simulink model "dynamic"  (R2023b)
settings: Solver=VariableStepAuto  StartTime=0.0  StopTime=5  MaxStep=1e-5  RelTol=1e-3
values from neighbouring files (symbols this model uses):
  phi0 = 0    [main.m]
  phidot0 = 0    [main.m]
  psif0 = 0    [main.m]
  psifdot0 = 0    [main.m]
  psir0 = 0    [main.m]
  psirdot0 = 0    [main.m]
  rho0 = 0    [main.m]
  rhodot0 = 0    [main.m]
  theta_dot_fl0 = xdot0*cos(car.toe.fl*pi/180)/car.tr.fl    [main.m]
  theta_dot_fr0 = xdot0*cos(car.toe.fr*pi/180)/car.tr.fr    [main.m]
  theta_dot_rl0 = xdot0*cos(car.toe.rl*pi/180)/car.tr.rl    [main.m]
  theta_dot_rr0 = xdot0*cos(car.toe.rr*pi/180)/car.tr.rr    [main.m]
  x0 = 0    [main.m]
  xdot0 = 10    [main.m]
  y0 = 0    [main.m]
  ydot0 = 0    [main.m]
  Zs0 = 0    [main.m]
  Zsdot0 = 0    [main.m]
  Zufl0 = 0    [main.m]
  Zufldot0 = 0    [main.m]
  Zufr0 = 0    [main.m]
  Zufrdot0 = 0    [main.m]
  Zurl0 = 0    [main.m]
  Zurldot0 = 0    [main.m]
  Zurr0 = 0    [main.m]
  Zurrdot0 = 0    [main.m]
undefined symbols (not defined in the file or in its folder): car
libraries: simulink x4, spsFirstOrderFilterLib x1
(part 2 of 2)

== system dynamic/Roll, Pitch, Heave/Unsprung/Unsprung rl ==
  Zf : Inport
  Z0 : Inport  Port=2
  Bus Creator : BusCreator  Inputs=3
  Bus Selector : BusSelector  OutputSignals=Zf_rl
  Bus Selector1 : BusSelector  OutputSignals=Z0_rl,Z0dot_rl
  Constant : Constant  Value=car.g
  Gain : Gain  Gain=car.K.t
  Gain1 : Gain  Gain=car.c.t
  Gain2 : Gain  Gain=1/car.murl
  Gain4 : Gain  Gain=car.murl
  Integrator : Integrator  InitialCondition=Zurldot0
  Integrator1 : Integrator  InitialCondition=Zurl0
  Minus : Sum  Inputs=----
  Minus1 : Sum  Inputs=+-
  Minus2 : Sum  Inputs=+-
  Minus3 : Sum
  Zu_rl : Outport
  FZ_rl : Outport  Port=2
  wires:
  Z0/1 -> Bus Selector1/1
  Zf/1 -> Bus Selector/1
  Bus Selector/1 -> Minus/1  "<Zf_rl>"
  Bus Selector1/1 -> Minus1/2  "<Z0_rl>"
  Minus1/1 -> Gain/1
  Gain/1 -> Minus/2, Minus3/1
  Bus Selector1/2 -> Minus2/2  "<Z0dot_rl>"
  Minus2/1 -> Gain1/1
  Gain1/1 -> Minus/3, Minus3/2
  Minus/1 -> Gain2/1
  Gain2/1 -> Bus Creator/3, Integrator/1  "Zurl_ddot"
  Integrator/1 -> Minus2/1, Bus Creator/2, Integrator1/1  "Zurl_dot"
  Integrator1/1 -> Minus1/1, Bus Creator/1  "Zurl"
  Bus Creator/1 -> Zu_rl/1  "Zu_rl"
  Gain4/1 -> Minus/4
  Constant/1 -> Gain4/1
  Minus3/1 -> FZ_rl/1  "FZ_rl"

== system dynamic/Roll, Pitch, Heave/Unsprung/Unsprung rr ==
  Zf : Inport
  Z0 : Inport  Port=2
  Bus Creator : BusCreator  Inputs=3
  Bus Selector : BusSelector  OutputSignals=Zf_rr
  Bus Selector1 : BusSelector  OutputSignals=Z0_rr,Z0dot_rr
  Constant : Constant  Value=car.g
  Gain : Gain  Gain=car.K.t
  Gain1 : Gain  Gain=car.c.t
  Gain2 : Gain  Gain=1/car.murr
  Gain4 : Gain  Gain=car.murr
  Integrator : Integrator  InitialCondition=Zurrdot0
  Integrator1 : Integrator  InitialCondition=Zurr0
  Minus : Sum  Inputs=----
  Minus1 : Sum  Inputs=+-
  Minus2 : Sum  Inputs=+-
  Minus3 : Sum
  Zu_rr : Outport
  FZ_rr : Outport  Port=2
  wires:
  Constant/1 -> Gain4/1
  Gain4/1 -> Minus/4
  Bus Creator/1 -> Zu_rr/1  "Zu_rr"
  Integrator1/1 -> Bus Creator/1, Minus1/1  "Zurr"
  Integrator/1 -> Integrator1/1, Bus Creator/2, Minus2/1  "Zurr_dot"
  Gain2/1 -> Integrator/1, Bus Creator/3  "Zurr_ddot"
  Minus/1 -> Gain2/1
  Gain1/1 -> Minus/3, Minus3/2
  Minus2/1 -> Gain1/1
  Bus Selector1/2 -> Minus2/2  "<Z0dot_rr>"
  Gain/1 -> Minus/2, Minus3/1
  Minus1/1 -> Gain/1
  Bus Selector1/1 -> Minus1/2  "<Z0_rr>"
  Bus Selector/1 -> Minus/1  "<Zf_rr>"
  Zf/1 -> Bus Selector/1
  Z0/1 -> Bus Selector1/1
  Minus3/1 -> FZ_rr/1  "FZ_rr"

== system dynamic/Roll, Pitch, Heave/Zs/Subsystem1 ==
  Zscgdot : Inport
  psi_fdot : Inport  Port=2
  psi_rdot : Inport  Port=3
  rhodot : Inport  Port=4
  Subsystem : Subsystem
  Subsystem1 : Subsystem
  Subsystem2 : Subsystem
  Subsystem3 : Subsystem
  Zsdot_fl : Outport
  Zsdot_fr : Outport  Port=2
  Zsdot_rl : Outport  Port=3
  Zsdot_rr : Outport  Port=4
  wires:
  Subsystem/1(Zsdot_fl) -> Zsdot_fl/1
  Subsystem2/1(Zsdot_rl) -> Zsdot_rl/1
  Subsystem1/1(Zsdot_fr) -> Zsdot_fr/1
  Zscgdot/1 -> Subsystem/1(Zscg), Subsystem1/1(Zscg), Subsystem2/1(Zscg), Subsystem3/1(Zscg)
  psi_rdot/1 -> Subsystem2/2(psi_r), Subsystem3/2(psi_r)
  rhodot/1 -> Subsystem3/3(rho), Subsystem2/3(rho), Subsystem/3(rho), Subsystem1/3(rho)
  psi_fdot/1 -> Subsystem1/2(psi_f), Subsystem/2(psi_f)
  Subsystem3/1(Zsdot_rr) -> Zsdot_rr/1

== system dynamic/Roll, Pitch, Heave/Zs/Subsystem4 ==
  Zscg : Inport
  psi_f : Inport  Port=2
  psi_r : Inport  Port=3
  rho : Inport  Port=4
  Subsystem : Subsystem
  Subsystem1 : Subsystem
  Subsystem2 : Subsystem
  Subsystem3 : Subsystem
  Zs_fl : Outport
  Zs_fr : Outport  Port=2
  Zs_rl : Outport  Port=3
  Zs_rr : Outport  Port=4
  wires:
  Subsystem3/1(Zs_rr) -> Zs_rr/1
  psi_f/1 -> Subsystem/2(psi_f), Subsystem1/2(psi_f)
  rho/1 -> Subsystem1/3(rho), Subsystem/3(rho), Subsystem2/3(rho), Subsystem3/3(rho)
  psi_r/1 -> Subsystem3/2(psi_r), Subsystem2/2(psi_r)
  Zscg/1 -> Subsystem3/1(Zscg), Subsystem2/1(Zscg), Subsystem1/1(Zscg), Subsystem/1(Zscg)
  Subsystem1/1(Zs_fr) -> Zs_fr/1
  Subsystem2/1(Zs_rl) -> Zs_rl/1
  Subsystem/1(Zs_fl) -> Zs_fl/1

== system dynamic/Roll, Pitch, Heave/corner forces/Zs_fl ==
  Zs : Inport
  Zu : Inport  Port=2
  M_roll : Inport  Port=3
  M_arb : Inport  Port=4
  Bus Selector : BusSelector  OutputSignals=M_inelas_f
  Bus Selector1 : BusSelector  OutputSignals=M_arb_f
  Bus Selector2 : BusSelector  OutputSignals=Zs_fl,Zsdot_fl
  Bus Selector3 : BusSelector  OutputSignals=Zu_fl.Zufl,Zu_fl.Zufl_dot
  Gain : Gain  Gain=car.K.fl
  Gain1 : Gain  Gain=car.c.fl
  Gain2 : Gain  Gain=car.r.fl/(car.r.fr*(car.r.fr+car.r.fl))
  Gain3 : Gain  Gain=car.r.fl/(car.r.fr*(car.r.fr+car.r.fl))
  Minus : Sum  Inputs=+-
  Minus1 : Sum  Inputs=+-
  Minus2 : Sum  Inputs=----
  Zf_fl : Outport
  wires:
  Minus1/1 -> Gain1/1
  Gain3/1 -> Minus2/4
  Gain/1 -> Minus2/1
  Gain1/1 -> Minus2/2
  Bus Selector1/1 -> Gain3/1  "<M_arb_f>"
  Gain2/1 -> Minus2/3
  M_roll/1 -> Bus Selector/1
  Bus Selector/1 -> Gain2/1  "<M_inelas_f>"
  Minus/1 -> Gain/1
  M_arb/1 -> Bus Selector1/1
  Minus2/1 -> Zf_fl/1  "Zf_fl"
  Zs/1 -> Bus Selector2/1
  Zu/1 -> Bus Selector3/1
  Bus Selector2/1 -> Minus/1  "<Zs_fl>"
  Bus Selector2/2 -> Minus1/1  "<Zsdot_fl>"
  Bus Selector3/1 -> Minus/2  "<Zufl>"
  Bus Selector3/2 -> Minus1/2  "<Zufl_dot>"

== system dynamic/Roll, Pitch, Heave/corner forces/Zs_fr ==
  M_roll : Inport
  M_arb : Inport  Port=2
  Zs : Inport  Port=3
  Zu : Inport  Port=4
  Bus Selector1 : BusSelector  OutputSignals=Zs_fr,Zsdot_fr
  Bus Selector2 : BusSelector  OutputSignals=M_inelas_f
  Bus Selector3 : BusSelector  OutputSignals=M_arb_f
  Bus Selector4 : BusSelector  OutputSignals=Zu_fr.Zufr,Zu_fr.Zufr_dot
  Gain4 : Gain  Gain=car.K.fr
  Gain5 : Gain  Gain=car.c.fr
  Gain6 : Gain  Gain=car.r.fr/(car.r.fl*(car.r.fr+car.r.fl))
  Gain7 : Gain  Gain=car.r.fr/(car.r.fl*(car.r.fr+car.r.fl))
  Minus3 : Sum  Inputs=+-
  Minus4 : Sum  Inputs=+-
  Minus5 : Sum  Inputs=--++
  Zf_fr : Outport
  wires:
  Bus Selector3/1 -> Gain7/1  "<M_arb_f>"
  Gain7/1 -> Minus5/4
  Minus3/1 -> Gain4/1
  Gain6/1 -> Minus5/3
  M_roll/1 -> Bus Selector2/1
  Gain5/1 -> Minus5/2
  Gain4/1 -> Minus5/1
  Bus Selector2/1 -> Gain6/1  "<M_inelas_f>"
  Minus4/1 -> Gain5/1
  M_arb/1 -> Bus Selector3/1
  Minus5/1 -> Zf_fr/1  "Zf_fr"
  Zs/1 -> Bus Selector1/1
  Zu/1 -> Bus Selector4/1
  Bus Selector1/1 -> Minus3/1  "<Zs_fr>"
  Bus Selector1/2 -> Minus4/1  "<Zsdot_fr>"
  Bus Selector4/1 -> Minus3/2  "<Zufr>"
  Bus Selector4/2 -> Minus4/2  "<Zufr_dot>"

== system dynamic/Roll, Pitch, Heave/corner forces/Zs_rl ==
  M_roll : Inport
  M_arb : Inport  Port=2
  Zs : Inport  Port=3
  Zu : Inport  Port=4
  Bus Selector1 : BusSelector  OutputSignals=Zs_rl,Zsdot_rl
  Bus Selector2 : BusSelector  OutputSignals=M_inelas_r
  Bus Selector3 : BusSelector  OutputSignals=M_arb_r
  Bus Selector4 : BusSelector  OutputSignals=Zu_rl.Zurl,Zu_rl.Zurl_dot
  Gain1 : Gain  Gain=car.r.rl/(car.r.rr*(car.r.rr+car.r.rl))
  Gain4 : Gain  Gain=car.K.rl
  Gain5 : Gain  Gain=car.c.rl
  Gain6 : Gain  Gain=car.r.rl/(car.r.rr*(car.r.rr+car.r.rl))
  Minus3 : Sum  Inputs=+-
  Minus4 : Sum  Inputs=+-
  Minus5 : Sum  Inputs=----
  Zf_rl : Outport
  wires:
  Minus5/1 -> Zf_rl/1  "Zf_rl"
  M_arb/1 -> Bus Selector3/1
  Minus4/1 -> Gain5/1
  Bus Selector2/1 -> Gain6/1  "<M_inelas_r>"
  Gain4/1 -> Minus5/1
  Gain5/1 -> Minus5/2
  M_roll/1 -> Bus Selector2/1
  Gain6/1 -> Minus5/3
  Minus3/1 -> Gain4/1
  Bus Selector3/1 -> Gain1/1  "<M_arb_r>"
  Gain1/1 -> Minus5/4
  Zs/1 -> Bus Selector1/1
  Zu/1 -> Bus Selector4/1
  Bus Selector1/1 -> Minus3/1  "<Zs_rl>"
  Bus Selector1/2 -> Minus4/1  "<Zsdot_rl>"
  Bus Selector4/1 -> Minus3/2  "<Zurl>"
  Bus Selector4/2 -> Minus4/2  "<Zurl_dot>"

== system dynamic/Roll, Pitch, Heave/corner forces/Zs_rr ==
  M_roll : Inport
  M_arb : Inport  Port=2
  Zs : Inport  Port=3
  Zu : Inport  Port=4
  Bus Selector1 : BusSelector  OutputSignals=Zs_rr,Zsdot_rr
  Bus Selector2 : BusSelector  OutputSignals=M_inelas_r
  Bus Selector3 : BusSelector  OutputSignals=M_arb_r
  Bus Selector4 : BusSelector  OutputSignals=Zu_rr.Zurr,Zu_rr.Zurr_dot
  Gain1 : Gain  Gain=car.r.rr/(car.r.rl*(car.r.rr+car.r.rl))
  Gain4 : Gain  Gain=car.K.rr
  Gain5 : Gain  Gain=car.c.rr
  Gain6 : Gain  Gain=car.r.rr/(car.r.rl*(car.r.rr+car.r.rl))
  Minus3 : Sum  Inputs=+-
  Minus4 : Sum  Inputs=+-
  Minus5 : Sum  Inputs=--++
  Zf_rr : Outport
  wires:
  Bus Selector3/1 -> Gain1/1  "<M_arb_r>"
  Minus3/1 -> Gain4/1
  Gain6/1 -> Minus5/3
  M_roll/1 -> Bus Selector2/1
  Gain5/1 -> Minus5/2
  Gain4/1 -> Minus5/1
  Bus Selector2/1 -> Gain6/1  "<M_inelas_r>"
  Minus4/1 -> Gain5/1
  M_arb/1 -> Bus Selector3/1
  Minus5/1 -> Zf_rr/1  "Zf_rr"
  Gain1/1 -> Minus5/4
  Zs/1 -> Bus Selector1/1
  Zu/1 -> Bus Selector4/1
  Bus Selector1/1 -> Minus3/1  "<Zs_rr>"
  Bus Selector1/2 -> Minus4/1  "<Zsdot_rr>"
  Bus Selector4/1 -> Minus3/2  "<Zurr>"
  Bus Selector4/2 -> Minus4/2  "<Zurr_dot>"

== system dynamic/Slip ratio/Xwdot/body to wheel frame ==
  xb : Inport
  delta : Inport  Port=2
  yb : Inport  Port=3
  Cos : Trigonometry  Operator=cos
  Cos1 : Trigonometry
  Gain : Gain  Gain=pi/180
  Minus : Sum
  Minus1 : Sum  Inputs=-+
  Product{,1..3} (4 alike) : Product
  xw : Outport
  yw : Outport  Port=2
  wires:
  Cos/1 -> Product3/2, Product/2
  Product2/1 -> Minus1/1
  Cos1/1 -> Product2/2, Product1/1
  yb/1 -> Product3/1, Product1/2
  Product1/1 -> Minus/2
  delta/1 -> Gain/1
  Minus/1 -> xw/1
  Product3/1 -> Minus1/2
  Product/1 -> Minus/1
  xb/1 -> Product2/1, Product/1
  Minus1/1 -> yw/1
  Gain/1 -> Cos1/1, Cos/1

== system dynamic/Slip ratio/Xwdot/body to wheel frame1 ==
  xb : Inport
  delta : Inport  Port=2
  yb : Inport  Port=3
  Cos : Trigonometry  Operator=cos
  Cos1 : Trigonometry
  Gain : Gain  Gain=pi/180
  Minus : Sum
  Minus1 : Sum  Inputs=-+
  Product{,1..3} (4 alike) : Product
  xw : Outport
  yw : Outport  Port=2
  wires:
  Minus1/1 -> yw/1
  xb/1 -> Product/1, Product2/1
  Product/1 -> Minus/1
  Product3/1 -> Minus1/2
  Minus/1 -> xw/1
  delta/1 -> Gain/1
  Product1/1 -> Minus/2
  yb/1 -> Product1/2, Product3/1
  Cos1/1 -> Product1/1, Product2/2
  Product2/1 -> Minus1/1
  Cos/1 -> Product/2, Product3/2
  Gain/1 -> Cos/1, Cos1/1

== system dynamic/Slip ratio/Xwdot/body to wheel frame2 ==
  xb : Inport
  delta : Inport  Port=2
  yb : Inport  Port=3
  Cos : Trigonometry  Operator=cos
  Cos1 : Trigonometry
  Gain : Gain  Gain=pi/180
  Minus : Sum
  Minus1 : Sum  Inputs=-+
  Product{,1..3} (4 alike) : Product
  xw : Outport
  yw : Outport  Port=2
  wires:
  Cos/1 -> Product3/2, Product/2
  Product2/1 -> Minus1/1
  Cos1/1 -> Product2/2, Product1/1
  yb/1 -> Product3/1, Product1/2
  Product1/1 -> Minus/2
  delta/1 -> Gain/1
  Minus/1 -> xw/1
  Product3/1 -> Minus1/2
  Product/1 -> Minus/1
  xb/1 -> Product2/1, Product/1
  Minus1/1 -> yw/1
  Gain/1 -> Cos1/1, Cos/1

== system dynamic/Slip ratio/Xwdot/body to wheel frame3 ==
  xb : Inport
  delta : Inport  Port=2
  yb : Inport  Port=3
  Cos : Trigonometry  Operator=cos
  Cos1 : Trigonometry
  Gain : Gain  Gain=pi/180
  Minus : Sum
  Minus1 : Sum  Inputs=-+
  Product{,1..3} (4 alike) : Product
  xw : Outport
  yw : Outport  Port=2
  wires:
  Minus1/1 -> yw/1
  xb/1 -> Product/1, Product2/1
  Product/1 -> Minus/1
  Product3/1 -> Minus1/2
  Minus/1 -> xw/1
  delta/1 -> Gain/1
  Product1/1 -> Minus/2
  yb/1 -> Product1/2, Product3/1
  Cos1/1 -> Product1/1, Product2/2
  Product2/1 -> Minus1/1
  Cos/1 -> Product/2, Product3/2
  Gain/1 -> Cos/1, Cos1/1

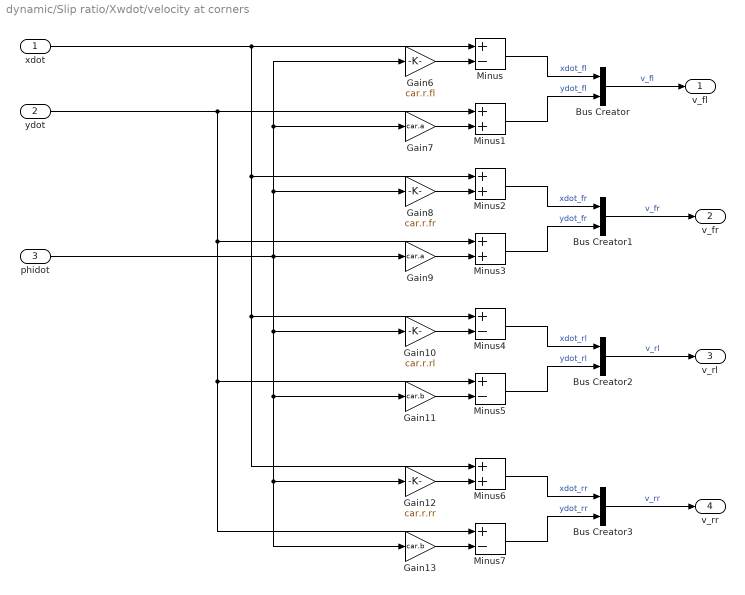
== system dynamic/Slip ratio/Xwdot/velocity at corners ==
  xdot : Inport
  ydot : Inport  Port=2
  phidot : Inport  Port=3
  Bus Creator{,1..3} (4 alike) : BusCreator  Inputs=2
  Gain10 : Gain  Gain=car.r.rl
  Gain11 : Gain  Gain=car.b
  Gain12 : Gain  Gain=car.r.rr
  Gain13 : Gain  Gain=car.b
  Gain6 : Gain  Gain=car.r.fl
  Gain7 : Gain  Gain=car.a
  Gain8 : Gain  Gain=car.r.fr
  Gain9 : Gain  Gain=car.a
  Minus{,4..5,7} (4 alike) : Sum  Inputs=+-
  Minus{1..3,6} (4 alike) : Sum
  v_fl : Outport
  v_fr : Outport  Port=2
  v_rl : Outport  Port=3
  v_rr : Outport  Port=4
  wires:
  ydot/1 -> Minus7/1, Minus5/1, Minus3/1, Minus1/1
  Gain8/1 -> Minus2/2
  Gain7/1 -> Minus1/2
  phidot/1 -> Gain7/1, Gain6/1, Gain8/1, Gain13/1, Gain12/1, Gain11/1, Gain10/1, Gain9/1
  Minus2/1 -> Bus Creator1/1  "xdot_fr"
  xdot/1 -> Minus6/1, Minus4/1, Minus2/1, Minus/1
  Minus1/1 -> Bus Creator/2  "ydot_fl"
  Gain9/1 -> Minus3/2
  Gain10/1 -> Minus4/2
  Gain11/1 -> Minus5/2
  Minus5/1 -> Bus Creator2/2  "ydot_rl"
  Minus4/1 -> Bus Creator2/1  "xdot_rl"
  Gain12/1 -> Minus6/2
  Minus7/1 -> Bus Creator3/2  "ydot_rr"
  Minus6/1 -> Bus Creator3/1  "xdot_rr"
  Gain13/1 -> Minus7/2
  Minus/1 -> Bus Creator/1  "xdot_fl"
  Gain6/1 -> Minus/2
  Minus3/1 -> Bus Creator1/2  "ydot_fr"
  Bus Creator2/1 -> v_rl/1  "v_rl"
  Bus Creator3/1 -> v_rr/1  "v_rr"
  Bus Creator1/1 -> v_fr/1  "v_fr"
  Bus Creator/1 -> v_fl/1  "v_fl"

== system dynamic/Roll, Pitch, Heave/Zs/Subsystem1/Subsystem ==
  Zscg : Inport
  psi_f : Inport  Port=2
  rho : Inport  Port=3
  Gain : Gain  Gain=car.r.fl
  Gain2 : Gain  Gain=car.a
  Minus : Sum  Inputs=++-
  Zsdot_fl : Outport
  wires:
  Zscg/1 -> Minus/1
  rho/1 -> Gain2/1
  Gain2/1 -> Minus/3
  Gain/1 -> Minus/2
  Minus/1 -> Zsdot_fl/1  "Zsdot_fl"
  psi_f/1 -> Gain/1

== system dynamic/Roll, Pitch, Heave/Zs/Subsystem1/Subsystem1 ==
  Zscg : Inport
  psi_f : Inport  Port=2
  rho : Inport  Port=3
  Gain : Gain  Gain=car.r.fr
  Gain2 : Gain  Gain=car.a
  Minus : Sum  Inputs=+--
  Zsdot_fr : Outport
  wires:
  psi_f/1 -> Gain/1
  Minus/1 -> Zsdot_fr/1  "Zsdot_fr"
  Gain/1 -> Minus/2
  Gain2/1 -> Minus/3
  rho/1 -> Gain2/1
  Zscg/1 -> Minus/1

== system dynamic/Roll, Pitch, Heave/Zs/Subsystem1/Subsystem2 ==
  Zscg : Inport
  psi_r : Inport  Port=2
  rho : Inport  Port=3
  Gain : Gain  Gain=car.r.rl
  Gain2 : Gain  Gain=car.b
  Minus : Sum  Inputs=+++
  Zsdot_rl : Outport
  wires:
  Zscg/1 -> Minus/1
  rho/1 -> Gain2/1
  Gain2/1 -> Minus/3
  Gain/1 -> Minus/2
  Minus/1 -> Zsdot_rl/1  "Zsdot_rl"
  psi_r/1 -> Gain/1

== system dynamic/Roll, Pitch, Heave/Zs/Subsystem1/Subsystem3 ==
  Zscg : Inport
  psi_r : Inport  Port=2
  rho : Inport  Port=3
  Gain : Gain  Gain=car.r.rr
  Gain2 : Gain  Gain=car.b
  Minus : Sum  Inputs=+-+
  Zsdot_rr : Outport
  wires:
  psi_r/1 -> Gain/1
  Minus/1 -> Zsdot_rr/1  "Zsdot_rr"
  Gain/1 -> Minus/2
  Gain2/1 -> Minus/3
  rho/1 -> Gain2/1
  Zscg/1 -> Minus/1

== system dynamic/Roll, Pitch, Heave/Zs/Subsystem4/Subsystem ==
  Zscg : Inport
  psi_f : Inport  Port=2
  rho : Inport  Port=3
  Gain : Gain  Gain=car.r.fl
  Gain2 : Gain  Gain=car.a
  Minus : Sum  Inputs=++-
  Zs_fl : Outport
  wires:
  Minus/1 -> Zs_fl/1  "Zs_fl"
  Gain/1 -> Minus/2
  Gain2/1 -> Minus/3
  rho/1 -> Gain2/1
  Zscg/1 -> Minus/1
  psi_f/1 -> Gain/1

== system dynamic/Roll, Pitch, Heave/Zs/Subsystem4/Subsystem1 ==
  Zscg : Inport
  psi_f : Inport  Port=2
  rho : Inport  Port=3
  Gain : Gain  Gain=car.r.fr
  Gain2 : Gain  Gain=car.a
  Minus : Sum  Inputs=+--
  Zs_fr : Outport
  wires:
  Zscg/1 -> Minus/1
  rho/1 -> Gain2/1
  Gain2/1 -> Minus/3
  Gain/1 -> Minus/2
  Minus/1 -> Zs_fr/1  "Zs_fr"
  psi_f/1 -> Gain/1

== system dynamic/Roll, Pitch, Heave/Zs/Subsystem4/Subsystem2 ==
  Zscg : Inport
  psi_r : Inport  Port=2
  rho : Inport  Port=3
  Gain : Gain  Gain=car.r.rl
  Gain2 : Gain  Gain=car.b
  Minus : Sum  Inputs=+++
  Zs_rl : Outport
  wires:
  psi_r/1 -> Gain/1
  Minus/1 -> Zs_rl/1  "Zs_rl"
  Gain/1 -> Minus/2
  Gain2/1 -> Minus/3
  rho/1 -> Gain2/1
  Zscg/1 -> Minus/1

== system dynamic/Roll, Pitch, Heave/Zs/Subsystem4/Subsystem3 ==
  Zscg : Inport
  psi_r : Inport  Port=2
  rho : Inport  Port=3
  Gain : Gain  Gain=car.r.rr
  Gain2 : Gain  Gain=car.b
  Minus : Sum  Inputs=+-+
  Zs_rr : Outport
  wires:
  Zscg/1 -> Minus/1
  rho/1 -> Gain2/1
  Gain2/1 -> Minus/3
  Gain/1 -> Minus/2
  Minus/1 -> Zs_rr/1  "Zs_rr"
  psi_r/1 -> Gain/1

== matlab function dynamic/tires/MATLAB Function ==
  data: SR_rr input; FXrr output; SR_rl input; SR_fr input; SR_fl input; SA_rr input; SA_rl input; SA_fr input; SA_fl input; FZ_rr input; FZ_rl input; FZ_fr input; FZ_fl input; tire parameter; FXrl output; FXfr output; FXfl output; FYrr output; FYrl output; FYfr output; FYfl output
function [FXrr,FXrl,FXfr,FXfl,FYrr,FYrl,FYfr,FYfl] = TireDynamics(SR_rr,SR_rl,SR_fr,SR_fl,SA_rr,SA_rl,SA_fr,SA_fl,FZ_rr,FZ_rl,FZ_fr,FZ_fl,tire)
% tire forces all in wheel frame
if FZ_rr <0
    FZ_rr =0;
end
if FZ_rl <0
    FZ_rl =0;
end
if FZ_fr <0
    FZ_fr =0;
end
if FZ_fl <0
    FZ_fl =0;
end

FX_rr = tire.scale*longforce(SR_rr,FZ_rr,tire.fz,tire.sr,tire.fx);
FX_rl = tire.scale*longforce(SR_rl,FZ_rl,tire.fz,tire.sr,tire.fx);
FX_fr = tire.scale*longforce(SR_fr,FZ_fr,tire.fz,tire.sr,tire.fx);
FX_fl = tire.scale*longforce(SR_fl,FZ_fl,tire.fz,tire.sr,tire.fx);

FY_rr = tire.scale*latforce(SA_rr,FZ_rr,tire.fz,tire.sa,tire.fy);
FY_rl = tire.scale*latforce(SA_rl,FZ_rl,tire.fz,tire.sa,tire.fy);
FY_fr = tire.scale*latforce(SA_fr,FZ_fr,tire.fz,tire.sa,tire.fy);
FY_fl = tire.scale*latforce(SA_fl,FZ_fl,tire.fz,tire.sa,tire.fy);

FXm_rr = tire.scale*interp1(tire.fz,tire.fx_max,FZ_rr);
FXm_rl = tire.scale*interp1(tire.fz,tire.fx_max,FZ_rl);
FXm_fr = tire.scale*interp1(tire.fz,tire.fx_max,FZ_fr);
FXm_fl = tire.scale*interp1(tire.fz,tire.fx_max,FZ_fl);

FXrr = sign(SR_rr)*FX_rr;
FXrl = sign(SR_rl)*FX_rl;
FXfr = sign(SR_fr)*FX_fr;
FXfl = sign(SR_fl)*FX_fl;

if FXm_rr == 0
    FYrr = sign(SA_rr)*FY_rr;
else
    FYrr = sign(SA_rr)*(sqrt((1-FX_rr^2/FXm_rr^2)*FY_rr^2));
end
if FXm_rl == 0
    FYrl = sign(SA_rl)*FY_rl;
else
    FYrl = sign(SA_rl)*(sqrt((1-FX_rl^2/FXm_rl^2)*FY_rl^2));
end
if FXm_fr == 0
    FYfr = sign(SA_fr)*FY_fr;
else
    FYfr = sign(SA_fr)*(sqrt((1-FX_fr^2/FXm_fr^2)*FY_fr^2));
end
if FXm_fl == 0
    FYfl = sign(SA_fl)*FY_fl;
else
    FYfl = sign(SA_fl)*(sqrt((1-FX_fl^2/FXm_fl^2)*FY_fl^2));
end
